simulink model "dataGen"  (R2019a)
settings: Solver=VariableStepAuto  StartTime=0.0  StopTime=10.0  RelTol=1e-3
settings Model: Creator=nhj94  LastModifiedBy=nhj94

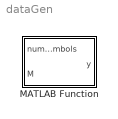
== system dataGen ==
  MATLAB Function : MATLAB Function  TreatAsAtomicUnit=on

== matlab function dataGen/MATLAB Function ==
  data: numSymbols input; y output; M input
function y = dataGen(numSymbols,M)
data = randi([0 M-1], numSymbols, 2);
y = data;
